simulink model "Wersja_z_02_01"  (R2018b)
settings: Solver=ode23s  StartTime=0  StopTime=5  MaxStep=0.01  RelTol=1e-06  AbsTol=1e-06
undefined symbols (not defined in the file or in its folder): Cpas, Cpat, Cpvn, Csas, Csat, Csvn, Lpas, Lpat, Lsas, Lsat, Rpar, Rpas, Rpat, Rpcp, Rpvn, Rsar, Rsas, Rsat, Rscp, Rsvn
settings Model: Creator=bartk  LastModifiedBy=bartk
settings DebuggingCC: LibraryContextMissingDiagnostic=none

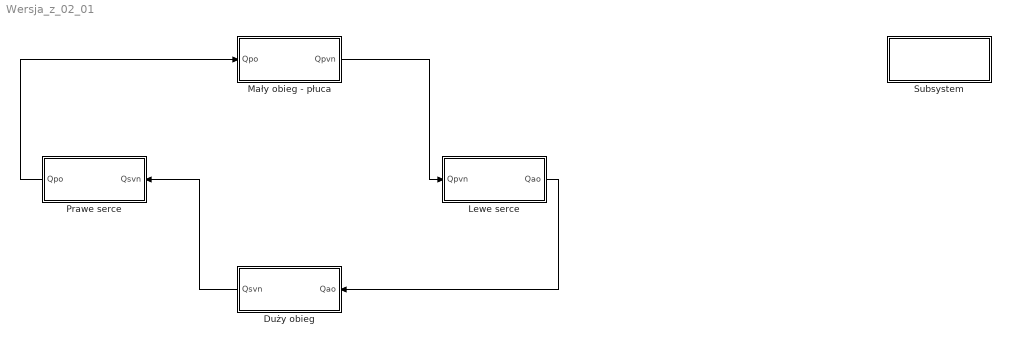
== system Wersja_z_02_01 ==
  "Duży obieg " : Subsystem
  "Lewe serce " : Subsystem
  "Mały obieg - płuca " : Subsystem
  "Prawe serce " : Subsystem
  Subsystem : Subsystem
  wires:
  "Duży obieg "/1(Qsvn) -> "Prawe serce "/1(Qsvn)
  "Prawe serce "/1(Qpo) -> "Mały obieg - płuca "/1(Qpo)
  "Lewe serce "/1(Qao) -> "Duży obieg "/1(Qao)
  "Mały obieg - płuca "/1(Qpvn) -> "Lewe serce "/1(Qpvn)

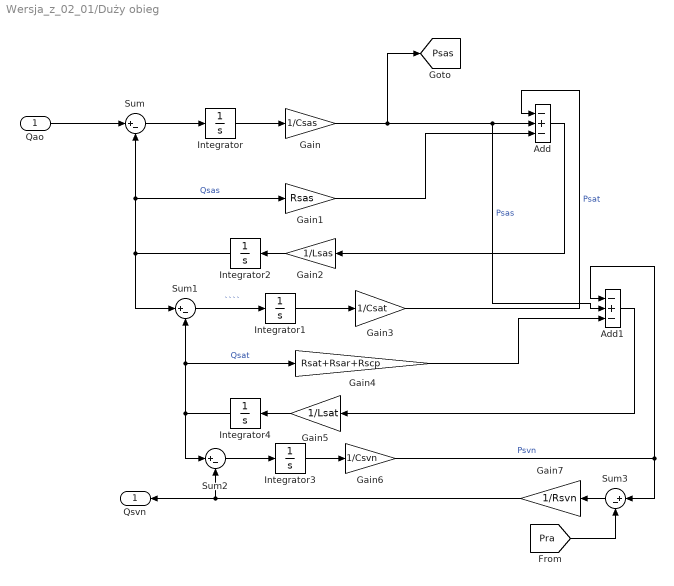
== system Wersja_z_02_01/Duży obieg  ==
  Qao : Inport
  Add : Sum  Inputs=-+-
  Add1 : Sum  Inputs=-+-
  Gain : Gain  Gain=1/Csas
  Gain1 : Gain  Gain=Rsas
  Gain2 : Gain  Gain=1/Lsas
  Gain3 : Gain  Gain=1/Csat
  Gain4 : Gain  Gain=Rsat+Rsar+Rscp
  Gain5 : Gain  Gain=1/Lsat
  Gain6 : Gain  Gain=1/Csvn
  Gain7 : Gain  Gain=1/Rsvn
  Integrator : Integrator  InitialCondition=100
  Integrator1 : Integrator  InitialCondition=100
  Integrator2 : Integrator
  Integrator3 : Integrator  InitialCondition=4
  Integrator4 : Integrator
  Sum{,1..3} (4 alike) : Sum  Inputs=|+-
  Qsvn : Outport
  tag scope: Psas=global
  wires:
  Qao/1 -> Sum/1
  Sum/1 -> Integrator/1
  Integrator/1 -> Gain/1
  Gain/1 -> [Psas], Add1/2, Add/2  "Psas"
  Gain1/1 -> Add/3
  Add/1 -> Gain2/1
  Sum1/1 -> Integrator1/1  "````"
  Gain3/1 -> Add/1  "Psat"
  Gain4/1 -> Add1/3
  Add1/1 -> Gain5/1
  Sum2/1 -> Integrator3/1
  Gain6/1 -> Add1/1, Sum3/1  "Psvn"
  Sum3/1 -> Gain7/1
  Gain7/1 -> Qsvn/1, Sum2/2
  [Pra] -> Sum3/2
  Gain5/1 -> Integrator4/1
  Gain2/1 -> Integrator2/1
  Integrator3/1 -> Gain6/1
  Integrator1/1 -> Gain3/1
  Integrator2/1 -> Sum1/1, Sum/2, Gain1/1  "Qsas"
  Integrator4/1 -> Gain4/1, Sum1/2, Sum2/1  "Qsat"

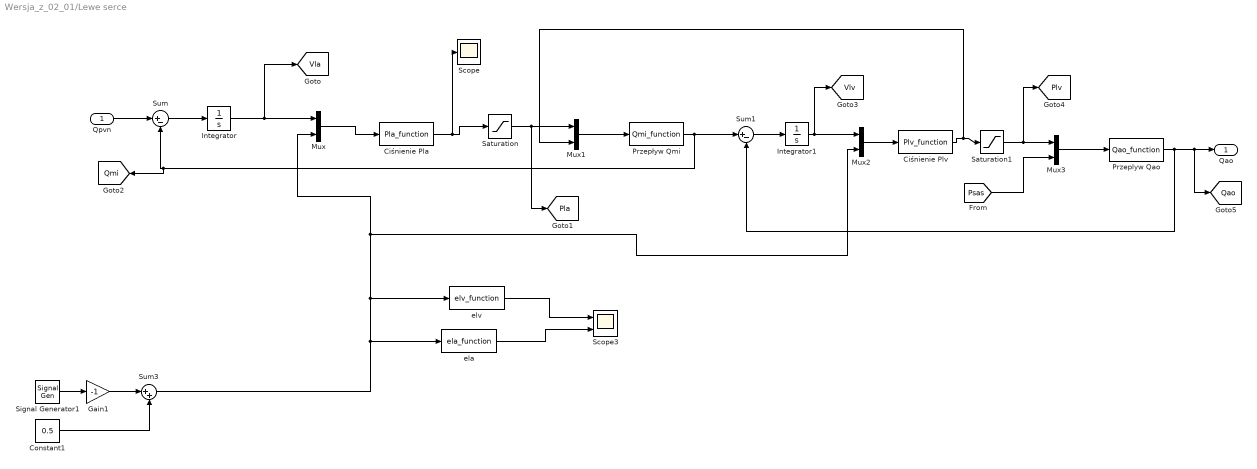
== system Wersja_z_02_01/Lewe serce  ==
  Qpvn : Inport
  Ciśnienie Pla : MATLABFcn  MATLABFcn=Pla_function
  "Ciśnienie Plv " : MATLABFcn  MATLABFcn=Plv_function
  Constant1 : Constant  Value=0.5
  Gain1 : Gain  Gain=-1
  Integrator : Integrator  InitialCondition=4
  Integrator1 : Integrator  InitialCondition=500
  Mux{,1..3} (4 alike) : Mux  Inputs=2
  Przeplyw Qao : MATLABFcn  MATLABFcn=Qao_function
  Przepływ Qmi : MATLABFcn  MATLABFcn=Qmi_function
  Saturation : Saturate  UpperLimit=inf  LowerLimit=0
  Saturation1 : Saturate  UpperLimit=inf  LowerLimit=0
  Scope : Scope
  Scope3 : Scope  NumInputPorts=2
  Signal Generator1 : SignalGenerator  WaveForm=sawtooth  Amplitude=0.5
  Sum : Sum  Inputs=|+-
  Sum1 : Sum  Inputs=|+-
  Sum3 : Sum  Inputs=|++
  ela : MATLABFcn  MATLABFcn=ela_function
  elv : MATLABFcn  MATLABFcn=elv_function
  Qao : Outport
  tag scope: Pla=global, Plv=global, Qao=global, Qmi=global, Vla=global, Vlv=global
  wires:
  Przepływ Qmi/1 -> Sum1/1, [Qmi], Sum/2
  Integrator1/1 -> Mux2/1, [Vlv]
  Sum3/1 -> elv/1, Mux2/2, Mux/2, ela/1
  Mux2/1 -> "Ciśnienie Plv "/1
  Mux3/1 -> Przeplyw Qao/1
  Przeplyw Qao/1 -> [Qao], Qao/1, Sum1/2
  Sum1/1 -> Integrator1/1
  [Psas] -> Mux3/2
  "Ciśnienie Plv "/1 -> Mux1/2, Saturation1/1
  Ciśnienie Pla/1 -> Scope/1, Saturation/1
  Mux1/1 -> Przepływ Qmi/1
  Mux/1 -> Ciśnienie Pla/1
  Integrator/1 -> Mux/1, [Vla]
  Sum/1 -> Integrator/1
  Saturation/1 -> [Pla], Mux1/1
  Qpvn/1 -> Sum/1
  Saturation1/1 -> [Plv], Mux3/1
  Signal Generator1/1 -> Gain1/1
  Constant1/1 -> Sum3/2
  Gain1/1 -> Sum3/1
  elv/1 -> Scope3/1
  ela/1 -> Scope3/2

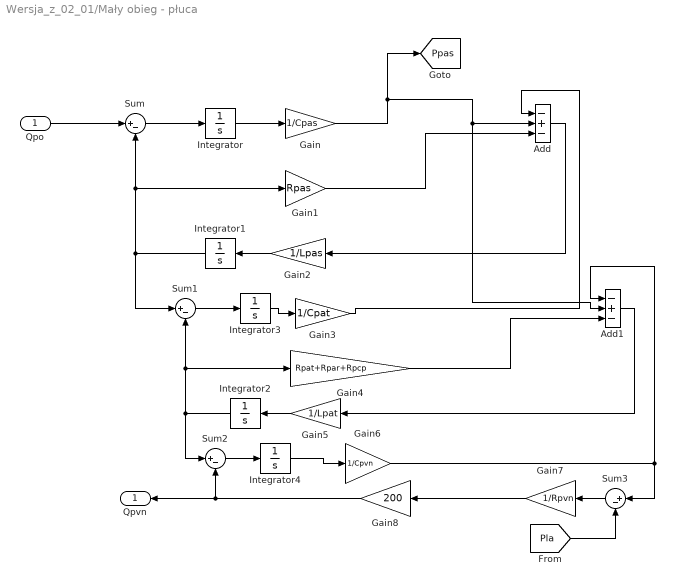
== system Wersja_z_02_01/Mały obieg - płuca  ==
  Qpo : Inport
  Add : Sum  Inputs=-+-
  Add1 : Sum  Inputs=-+-
  Gain : Gain  Gain=1/Cpas
  Gain1 : Gain  Gain=Rpas
  Gain2 : Gain  Gain=1/Lpas
  Gain3 : Gain  Gain=1/Cpat
  Gain4 : Gain  Gain=Rpat+Rpar+Rpcp
  Gain5 : Gain  Gain=1/Lpat
  Gain6 : Gain  Gain=1/Cpvn
  Gain7 : Gain  Gain=1/Rpvn
  Gain8 : Gain  Gain=200
  Integrator : Integrator  InitialCondition=30
  Integrator1 : Integrator
  Integrator2 : Integrator
  Integrator3 : Integrator  InitialCondition=30
  Integrator4 : Integrator  InitialCondition=8
  Sum{,1..3} (4 alike) : Sum  Inputs=|+-
  Qpvn : Outport
  tag scope: Ppas=global
  wires:
  Gain6/1 -> Add1/1, Sum3/1
  [Pla] -> Sum3/2
  Sum2/1 -> Integrator4/1
  Gain7/1 -> Gain8/1
  Gain3/1 -> Add/1
  Integrator/1 -> Gain/1
  Add/1 -> Gain2/1
  Gain5/1 -> Integrator2/1
  Gain/1 -> [Ppas], Add1/2, Add/2
  Add1/1 -> Gain5/1
  Gain4/1 -> Add1/3
  Sum1/1 -> Integrator3/1
  Sum/1 -> Integrator/1
  Qpo/1 -> Sum/1
  Sum3/1 -> Gain7/1
  Gain1/1 -> Add/3
  Gain2/1 -> Integrator1/1
  Integrator2/1 -> Sum1/2, Gain4/1, Sum2/1
  Integrator1/1 -> Sum1/1, Sum/2, Gain1/1
  Integrator3/1 -> Gain3/1
  Integrator4/1 -> Gain6/1
  Gain8/1 -> Qpvn/1, Sum2/2

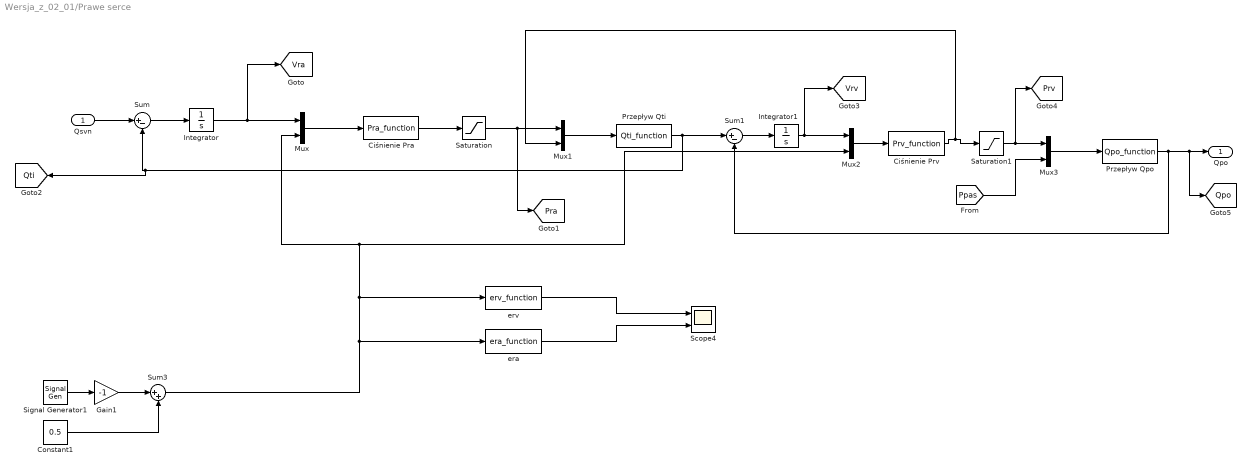
== system Wersja_z_02_01/Prawe serce  ==
  Qsvn : Inport
  "Ciśnienie Pra " : MATLABFcn  MATLABFcn=Pra_function
  Ciśnienie Prv : MATLABFcn  MATLABFcn=Prv_function
  Constant1 : Constant  Value=0.5
  Gain1 : Gain  Gain=-1
  Integrator : Integrator  InitialCondition=4
  Integrator1 : Integrator  InitialCondition=400
  Mux{,1..3} (4 alike) : Mux  Inputs=2
  Przepływ Qpo : MATLABFcn  MATLABFcn=Qpo_function
  Przepływ Qti : MATLABFcn  MATLABFcn=Qti_function
  Saturation : Saturate  UpperLimit=inf  LowerLimit=0
  Saturation1 : Saturate  UpperLimit=inf  LowerLimit=0
  Scope4 : Scope  NumInputPorts=2
  Signal Generator1 : SignalGenerator  WaveForm=sawtooth  Amplitude=0.5
  Sum : Sum  Inputs=|+-
  Sum1 : Sum  Inputs=|+-
  Sum3 : Sum  Inputs=|++
  era : MATLABFcn  MATLABFcn=era_function
  erv : MATLABFcn  MATLABFcn=erv_function
  Qpo : Outport
  tag scope: Pra=global, Prv=global, Qpo=global, Qti=global, Vra=global, Vrv=global
  wires:
  Qsvn/1 -> Sum/1
  Sum/1 -> Integrator/1
  Integrator/1 -> Mux/1, [Vra]
  Mux/1 -> "Ciśnienie Pra "/1
  "Ciśnienie Pra "/1 -> Saturation/1
  Mux1/1 -> Przepływ Qti/1
  Przepływ Qti/1 -> Sum1/1, [Qti], Sum/2
  Sum1/1 -> Integrator1/1
  Integrator1/1 -> Mux2/1, [Vrv]
  Mux2/1 -> Ciśnienie Prv/1
  Ciśnienie Prv/1 -> Saturation1/1, Mux1/2
  [Ppas] -> Mux3/2
  Mux3/1 -> Przepływ Qpo/1
  Przepływ Qpo/1 -> [Qpo], Qpo/1, Sum1/2
  Sum3/1 -> erv/1, Mux/2, Mux2/2, era/1
  Constant1/1 -> Sum3/2
  Signal Generator1/1 -> Gain1/1
  Gain1/1 -> Sum3/1
  Saturation/1 -> [Pra], Mux1/1
  Saturation1/1 -> [Prv], Mux3/1
  erv/1 -> Scope4/1
  era/1 -> Scope4/2

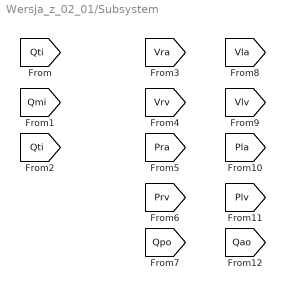
== system Wersja_z_02_01/Subsystem ==
